simulink model "abslut10_fixpt8_32"  (R2021b)
settings: Solver=VariableStepAuto  StartTime=0.0  StopTime=99  RelTol=1e-3
undefined symbols (not defined in the file or in its folder): figd2104, xcu250
libraries: hdlBasic x2875, vmcUtilities x1
(part 12 of 24)

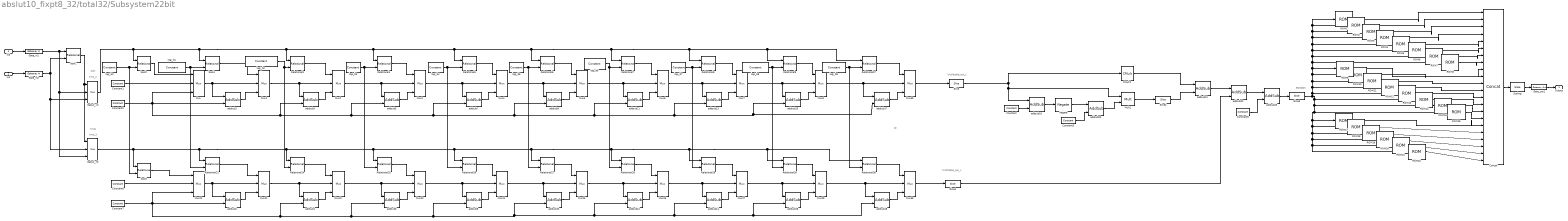
== system abslut10_fixpt8_32/total32/Subsystem22bit ==
  note: 10
  note: tiisai
  note: ooki
  note: 55no6bit
  note: tmp_2
  note: tmp_3
  note: truthtable_out_x
  note: truthtable_out_y
  In3 : Inport
  In4 : Inport  Port=2
  CMult1 : hdlBasic/CMult  const=10  gui_display_data_type=Fixed-point  const_n_bits=4  const_bin_pt=0  float_type=Single  exp_bits=8  fraction_bits=24  en=off  latency=0  precision=Full  arith_type="Signed  (2's comp)"  n_bits=16  bin_pt=14  quantization=Truncate  overflow=Wrap  use_behavioral_HDL=off  mem_type=Distributed RAM  pipeline=off  XmcBlockStatus=1  maskContainerNames=tabcontainer1  block_type=cmult  block_config=sysgen:CMult_config
      settings: infoedit=[]
  Concat : hdlBasic/Concat  num_inputs=22  XmcBlockStatus=1  maskContainerNames=group1  block_type=concat  block_config=sysgen:Concat_config
  Constant : hdlBasic/Constant  const=1.0  gui_display_data_type=Fixed-point  arith_type=Unsigned  n_bits=1  bin_pt=0  preci_type=Single  exp_width=8  frac_width=24  explicit_period=on  period=1  XmcBlockStatus=1  maskContainerNames=tabcontainer1  block_type=constant  block_config=sysgen:Constant_config
  Constant1 : hdlBasic/Constant  const=0  gui_display_data_type=Fixed-point  arith_type=Unsigned  n_bits=4  bin_pt=0  preci_type=Single  exp_width=8  frac_width=24  explicit_period=on  period=1  XmcBlockStatus=1  maskContainerNames=tabcontainer1  block_type=constant  block_config=sysgen:Constant_config
  Constant2 : hdlBasic/Constant  const=1  gui_display_data_type=Fixed-point  arith_type=Unsigned  n_bits=4  bin_pt=0  preci_type=Single  exp_width=8  frac_width=24  explicit_period=on  period=1  XmcBlockStatus=1  maskContainerNames=tabcontainer1  block_type=constant  block_config=sysgen:Constant_config
  Constant3 : hdlBasic/Constant  const=18  gui_display_data_type=Fixed-point  arith_type=Unsigned  n_bits=6  bin_pt=0  preci_type=Single  exp_width=8  frac_width=24  explicit_period=on  period=1  XmcBlockStatus=1  maskContainerNames=tabcontainer1  block_type=constant  block_config=sysgen:Constant_config
  Constant5 : hdlBasic/Constant  const=1.0  gui_display_data_type=Fixed-point  arith_type=Unsigned  n_bits=10  bin_pt=0  preci_type=Single  exp_width=8  frac_width=24  explicit_period=on  period=1  XmcBlockStatus=1  maskContainerNames=tabcontainer1  block_type=constant  block_config=sysgen:Constant_config
  Constant6 : hdlBasic/Constant  const=0  gui_display_data_type=Fixed-point  arith_type=Unsigned  n_bits=4  bin_pt=0  preci_type=Single  exp_width=8  frac_width=24  explicit_period=on  period=1  XmcBlockStatus=1  maskContainerNames=tabcontainer1  block_type=constant  block_config=sysgen:Constant_config
  Constant7 : hdlBasic/Constant  const=1  gui_display_data_type=Fixed-point  arith_type=Unsigned  n_bits=4  bin_pt=0  preci_type=Single  exp_width=8  frac_width=24  explicit_period=on  period=1  XmcBlockStatus=1  maskContainerNames=tabcontainer1  block_type=constant  block_config=sysgen:Constant_config
  Gate_In1 : hdlBasic/Gateway In  gui_display_data_type=Fixed-point  arith_type=Signed (2's comp)  n_bits=22  bin_pt=20  preci_type=Double  exp_width=8  frac_width=24  rows=1  columns=1  quantization="Round  (unbiased: +/- Inf)"  overflow=Saturate  period=1  UseAsADC=off  ADCChannel='1'  interface=None  automatic_assignment=on  address_offset=hex2dec('00')  intf_name=''  intf_description=''  default_value=0  timing_constraint=None  locs_specified=off  LOCs={}  io_standard={}  inherit_from_input=off  hdl_port=on  XmcBlockStatus=1  maskContainerNames=group4  block_type=gatewayin  block_config=sysgen:gateway_in_config  block_width_w=590  block_height_w=620  block_width=640  block_height=850
  Gate_In2 : hdlBasic/Gateway In  gui_display_data_type=Fixed-point  arith_type=Signed (2's comp)  n_bits=22  bin_pt=20  preci_type=Double  exp_width=8  frac_width=24  rows=1  columns=1  quantization="Round  (unbiased: +/- Inf)"  overflow=Saturate  period=1  UseAsADC=off  ADCChannel='1'  interface=None  automatic_assignment=on  address_offset=hex2dec('00')  intf_name=''  intf_description=''  default_value=0  timing_constraint=None  locs_specified=off  LOCs={}  io_standard={}  inherit_from_input=off  hdl_port=on  XmcBlockStatus=1  maskContainerNames=group4  block_type=gatewayin  block_config=sysgen:gateway_in_config  block_width_w=590  block_height_w=620  block_width=640  block_height=850
  Gate_out1 : hdlBasic/Gateway Out  inherit_from_input=off  hdl_port=on  rows=1  columns=1  UseAsDAC=off  DACChannel='1'  interface=None  automatic_assignment=on  address_offset=hex2dec('00')  intf_name=''  intf_description=''  timing_constraint=None  locs_specified=off  LOCs={}  io_standard={}  XmcBlockStatus=1  maskContainerNames=group4  block_type=gatewayout  block_config=sysgen:gateway_out_config  block_width_w=590  block_height_w=620  block_width=620  block_height=750
  Mult1 : hdlBasic/Mult  precision=Full  arith_type="Signed  (2's comp)"  n_bits=30  bin_pt=16  quantization="Round  (unbiased: +/- Inf)"  overflow=Saturate  en=off  latency=0  use_behavioral_HDL=off  opt=Area  use_embedded=off  optimum_pipeline=off  pipeline=on  use_rpm=on  placement_style=Triangular  XmcBlockStatus=1  maskContainerNames=group1  block_type=mult  block_config=sysgen:Mult_config
  Mux{,1..8,20..28,38..39} (20 alike) : hdlBasic/Mux  inputs=2  en=off  latency=0  precision=Full  arith_type=Unsigned  n_bits=16  bin_pt=14  quantization=Truncate  overflow=Wrap  XmcBlockStatus=1  maskContainerNames=tabcontainer1  block_type=mux  block_config=sysgen:Mux_config
  Negate : hdlBasic/Negate  precision=Full  arith_type=Unsigned  n_bits=16  bin_pt=14  quantization=Truncate  overflow=Wrap  en=off  latency=0  XmcBlockStatus=1  maskContainerNames=tabcontainer1  block_type=negate  block_config=sysgen:Negate_config
  ROM1 : hdlBasic/ROM  depth=55  initVector=[1,1,1,1,0,0,1,0,0,0,1,0,0,0,0,1,0,0,0,0,0,1,0,0,0,0,0,0,1,0,0,0,0,0,0,0,1,1,0,0,0,0,0,0,1,1,1,1,1,1,1,1,1,1,1]  distributed_mem=Distributed memory  rst=off  init_reg=0  en=off  latency=0  gui_display_data_type=Boolean  arith_type=Boolean  n_bits=2  bin_pt=0  preci_type=Double  exp_width=8  frac_width=24  optimize=Speed  use_rpm=on  simulation_type=fast_sim  XmcBlockStatus=1  maskContainerNames=tabcontainer1  block_type=sprom  block_config=sysgen:SPROM_config
  ROM10 : hdlBasic/ROM  depth=55  initVector=[0,0,1,1,1,0,1,1,1,1,1,0,0,1,0,1,0,0,1,0,0,1,1,1,1,1,1,1,1,1,0,1,0,0,1,0,0,1,1,1,0,0,1,1,1,0,0,1,1,1,1,1,1,0,0]  distributed_mem=Distributed memory  rst=off  init_reg=0  en=off  latency=0  gui_display_data_type=Boolean  arith_type=Boolean  n_bits=2  bin_pt=0  preci_type=Double  exp_width=8  frac_width=24  optimize=Speed  use_rpm=on  simulation_type=fast_sim  XmcBlockStatus=1  maskContainerNames=tabcontainer1  block_type=sprom  block_config=sysgen:SPROM_config
  ROM11 : hdlBasic/ROM  depth=55  initVector=[0,1,0,1,0,0,1,0,1,0,0,0,0,1,0,0,0,0,1,0,0,1,0,1,0,1,1,0,1,0,0,1,0,0,1,0,1,0,0,0,0,0,0,0,0,0,1,1,1,0,0,1,1,1,0]  distributed_mem=Distributed memory  rst=off  init_reg=0  en=off  latency=0  gui_display_data_type=Boolean  arith_type=Boolean  n_bits=2  bin_pt=0  preci_type=Double  exp_width=8  frac_width=24  optimize=Speed  use_rpm=on  simulation_type=fast_sim  XmcBlockStatus=1  maskContainerNames=tabcontainer1  block_type=sprom  block_config=sysgen:SPROM_config
  ROM12 : hdlBasic/ROM  depth=55  initVector=[0,0,0,0,1,1,0,1,0,1,0,1,0,1,1,0,1,0,1,1,1,0,1,0,1,1,1,1,0,1,1,0,0,0,0,1,0,0,1,1,1,1,1,1,0,0,0,0,0,0,0,0,0,0,0]  distributed_mem=Distributed memory  rst=off  init_reg=0  en=off  latency=0  gui_display_data_type=Boolean  arith_type=Boolean  n_bits=2  bin_pt=0  preci_type=Double  exp_width=8  frac_width=24  optimize=Speed  use_rpm=on  simulation_type=fast_sim  XmcBlockStatus=1  maskContainerNames=tabcontainer1  block_type=sprom  block_config=sysgen:SPROM_config
  ROM13 : hdlBasic/ROM  depth=55  initVector=[0,1,1,1,1,0,1,0,1,0,1,0,0,1,1,1,0,0,1,1,1,1,0,1,0,1,1,0,1,1,0,1,0,0,1,0,1,1,1,0,0,0,0,1,1,0,1,1,1,1,1,1,1,1,0]  distributed_mem=Distributed memory  rst=off  init_reg=0  en=off  latency=0  gui_display_data_type=Boolean  arith_type=Boolean  n_bits=2  bin_pt=0  preci_type=Double  exp_width=8  frac_width=24  optimize=Speed  use_rpm=on  simulation_type=fast_sim  XmcBlockStatus=1  maskContainerNames=tabcontainer1  block_type=sprom  block_config=sysgen:SPROM_config
  ROM14 : hdlBasic/ROM  depth=55  initVector=[1,0,0,1,0,0,1,0,1,1,0,0,1,0,1,0,0,1,0,1,1,1,0,1,1,0,0,1,1,0,0,1,1,1,1,0,0,0,0,0,0,0,0,0,0,1,0,1,1,0,0,1,1,0,1]  distributed_mem=Distributed memory  rst=off  init_reg=0  en=off  latency=0  gui_display_data_type=Boolean  arith_type=Boolean  n_bits=2  bin_pt=0  preci_type=Double  exp_width=8  frac_width=24  optimize=Speed  use_rpm=on  simulation_type=fast_sim  XmcBlockStatus=1  maskContainerNames=tabcontainer1  block_type=sprom  block_config=sysgen:SPROM_config
  ROM15 : hdlBasic/ROM  depth=55  initVector=[0,0,1,0,0,0,0,0,0,1,0,0,0,0,0,0,0,0,0,0,0,0,0,0,1,0,0,1,0,0,0,0,0,0,0,0,0,1,0,0,0,0,0,0,1,0,0,0,0,0,0,0,0,0,0]  distributed_mem=Distributed memory  rst=off  init_reg=0  en=off  latency=0  gui_display_data_type=Boolean  arith_type=Boolean  n_bits=2  bin_pt=0  preci_type=Double  exp_width=8  frac_width=24  optimize=Speed  use_rpm=on  simulation_type=fast_sim  XmcBlockStatus=1  maskContainerNames=tabcontainer1  block_type=sprom  block_config=sysgen:SPROM_config
  ROM16 : hdlBasic/ROM  depth=55  initVector=[0,0,0,1,0,0,0,0,1,0,1,0,0,1,0,1,0,0,1,0,0,0,0,1,0,1,1,0,1,0,0,1,0,0,1,0,0,0,0,0,0,0,0,0,0,0,0,1,0,1,1,0,1,0,0]  distributed_mem=Distributed memory  rst=off  init_reg=0  en=off  latency=0  gui_display_data_type=Boolean  arith_type=Boolean  n_bits=2  bin_pt=0  preci_type=Double  exp_width=8  frac_width=24  optimize=Speed  use_rpm=on  simulation_type=fast_sim  XmcBlockStatus=1  maskContainerNames=tabcontainer1  block_type=sprom  block_config=sysgen:SPROM_config
  ROM17 : hdlBasic/ROM  depth=55  initVector=[1,1,1,0,0,1,1,0,1,1,1,1,1,1,1,1,1,1,1,1,1,1,0,1,1,1,1,1,0,0,1,1,1,1,1,1,1,1,0,0,1,1,0,0,1,1,1,0,1,1,1,1,0,1,1]  distributed_mem=Distributed memory  rst=off  init_reg=0  en=off  latency=0  gui_display_data_type=Boolean  arith_type=Boolean  n_bits=2  bin_pt=0  preci_type=Double  exp_width=8  frac_width=24  optimize=Speed  use_rpm=on  simulation_type=fast_sim  XmcBlockStatus=1  maskContainerNames=tabcontainer1  block_type=sprom  block_config=sysgen:SPROM_config
  ROM18 : hdlBasic/ROM  depth=55  initVector=[1,0,1,0,0,1,0,0,1,1,0,1,1,0,1,0,1,1,0,1,1,0,0,1,1,0,0,1,0,0,1,1,1,1,1,1,0,1,0,0,1,1,0,0,1,1,0,0,0,0,0,0,0,0,1]  distributed_mem=Distributed memory  rst=off  init_reg=0  en=off  latency=0  gui_display_data_type=Boolean  arith_type=Boolean  n_bits=2  bin_pt=0  preci_type=Double  exp_width=8  frac_width=24  optimize=Speed  use_rpm=on  simulation_type=fast_sim  XmcBlockStatus=1  maskContainerNames=tabcontainer1  block_type=sprom  block_config=sysgen:SPROM_config
  ROM19 : hdlBasic/ROM  depth=55  initVector=[1,0,1,1,0,1,0,1,0,1,1,1,1,0,1,1,1,1,0,1,1,0,1,0,1,0,0,1,1,0,1,0,1,1,0,1,0,1,0,1,1,1,1,0,1,1,0,1,0,1,1,0,1,0,1]  distributed_mem=Distributed memory  rst=off  init_reg=0  en=off  latency=0  gui_display_data_type=Boolean  arith_type=Boolean  n_bits=2  bin_pt=0  preci_type=Double  exp_width=8  frac_width=24  optimize=Speed  use_rpm=on  simulation_type=fast_sim  XmcBlockStatus=1  maskContainerNames=tabcontainer1  block_type=sprom  block_config=sysgen:SPROM_config
  ROM2 : hdlBasic/ROM  depth=55  initVector=[0,0,0,0,1,1,0,1,1,0,0,1,1,0,0,0,1,1,0,0,0,0,1,1,0,0,0,0,0,1,1,1,1,1,1,1,0,0,1,1,1,1,1,1,0,0,0,0,0,0,0,0,0,0,0]  distributed_mem=Distributed memory  rst=off  init_reg=0  en=off  latency=0  gui_display_data_type=Boolean  arith_type=Boolean  n_bits=2  bin_pt=0  preci_type=Double  exp_width=8  frac_width=24  optimize=Speed  use_rpm=on  simulation_type=fast_sim  XmcBlockStatus=1  maskContainerNames=tabcontainer1  block_type=sprom  block_config=sysgen:SPROM_config
  ROM20 : hdlBasic/ROM  depth=55  initVector=[1,0,1,1,1,1,0,0,1,1,0,1,1,0,1,0,1,1,0,1,1,0,0,1,1,0,0,1,1,1,1,1,1,1,1,1,0,1,1,0,1,1,0,1,1,1,0,1,0,0,0,0,1,0,1]  distributed_mem=Distributed memory  rst=off  init_reg=0  en=off  latency=0  gui_display_data_type=Boolean  arith_type=Boolean  n_bits=2  bin_pt=0  preci_type=Double  exp_width=8  frac_width=24  optimize=Speed  use_rpm=on  simulation_type=fast_sim  XmcBlockStatus=1  maskContainerNames=tabcontainer1  block_type=sprom  block_config=sysgen:SPROM_config
  ROM21 : hdlBasic/ROM  depth=55  initVector=[0,0,0,1,1,1,0,1,1,1,0,1,0,0,1,0,1,0,0,1,1,0,1,1,1,0,0,1,1,1,1,1,0,0,1,1,0,0,1,1,1,1,1,1,0,0,0,1,0,0,0,0,1,0,0]  distributed_mem=Distributed memory  rst=off  init_reg=0  en=off  latency=0  gui_display_data_type=Boolean  arith_type=Boolean  n_bits=2  bin_pt=0  preci_type=Double  exp_width=8  frac_width=24  optimize=Speed  use_rpm=on  simulation_type=fast_sim  XmcBlockStatus=1  maskContainerNames=tabcontainer1  block_type=sprom  block_config=sysgen:SPROM_config
  ROM22 : hdlBasic/ROM  depth=55  initVector=[0,1,1,1,1,0,0,1,0,0,1,0,1,0,1,1,0,1,0,1,1,0,1,0,0,0,0,0,1,1,0,0,1,1,0,0,1,1,1,1,0,0,1,1,1,0,1,1,0,1,1,0,1,1,0]  distributed_mem=Distributed memory  rst=off  init_reg=0  en=off  latency=0  gui_display_data_type=Boolean  arith_type=Boolean  n_bits=2  bin_pt=0  preci_type=Double  exp_width=8  frac_width=24  optimize=Speed  use_rpm=on  simulation_type=fast_sim  XmcBlockStatus=1  maskContainerNames=tabcontainer1  block_type=sprom  block_config=sysgen:SPROM_config
  ROM3 : hdlBasic/ROM  depth=55  initVector=[1,1,0,0,1,1,0,1,0,1,0,1,0,1,0,0,1,0,1,0,0,0,1,0,1,1,1,1,0,1,1,0,0,0,0,1,1,0,1,1,1,1,1,1,0,1,1,0,0,0,0,0,0,1,1]  distributed_mem=Distributed memory  rst=off  init_reg=0  en=off  latency=0  gui_display_data_type=Boolean  arith_type=Boolean  n_bits=2  bin_pt=0  preci_type=Double  exp_width=8  frac_width=24  optimize=Speed  use_rpm=on  simulation_type=fast_sim  XmcBlockStatus=1  maskContainerNames=tabcontainer1  block_type=sprom  block_config=sysgen:SPROM_config
  ROM4 : hdlBasic/ROM  depth=55  initVector=[1,0,0,1,1,0,0,0,1,1,0,0,0,0,1,0,0,0,0,1,1,0,0,1,1,0,0,1,1,1,0,1,0,0,1,0,0,0,1,0,0,0,0,1,0,1,0,1,0,0,0,0,1,0,1]  distributed_mem=Distributed memory  rst=off  init_reg=0  en=off  latency=0  gui_display_data_type=Boolean  arith_type=Boolean  n_bits=2  bin_pt=0  preci_type=Double  exp_width=8  frac_width=24  optimize=Speed  use_rpm=on  simulation_type=fast_sim  XmcBlockStatus=1  maskContainerNames=tabcontainer1  block_type=sprom  block_config=sysgen:SPROM_config
  ROM5 : hdlBasic/ROM  depth=55  initVector=[0,0,1,0,1,0,0,1,0,1,0,0,1,1,0,0,0,1,1,0,0,0,1,0,1,1,1,1,0,1,0,0,1,1,0,0,0,1,1,1,0,0,1,1,1,0,0,0,0,0,0,0,0,0,0]  distributed_mem=Distributed memory  rst=off  init_reg=0  en=off  latency=0  gui_display_data_type=Boolean  arith_type=Boolean  n_bits=2  bin_pt=0  preci_type=Double  exp_width=8  frac_width=24  optimize=Speed  use_rpm=on  simulation_type=fast_sim  XmcBlockStatus=1  maskContainerNames=tabcontainer1  block_type=sprom  block_config=sysgen:SPROM_config
  ROM6 : hdlBasic/ROM  depth=55  initVector=[1,0,1,0,0,1,1,1,0,1,0,1,0,1,1,0,1,0,1,1,1,1,1,0,1,1,1,1,0,0,1,0,0,0,0,1,0,1,0,1,1,1,1,0,1,1,0,0,1,0,0,1,0,0,1]  distributed_mem=Distributed memory  rst=off  init_reg=0  en=off  latency=0  gui_display_data_type=Boolean  arith_type=Boolean  n_bits=2  bin_pt=0  preci_type=Double  exp_width=8  frac_width=24  optimize=Speed  use_rpm=on  simulation_type=fast_sim  XmcBlockStatus=1  maskContainerNames=tabcontainer1  block_type=sprom  block_config=sysgen:SPROM_config
  ROM7 : hdlBasic/ROM  depth=55  initVector=[0,1,0,1,1,0,1,0,1,0,0,0,0,0,0,0,0,0,0,0,0,1,0,1,0,0,0,0,1,1,0,1,0,0,1,0,1,0,1,0,0,0,0,1,0,0,1,1,1,0,0,1,1,1,0]  distributed_mem=Distributed memory  rst=off  init_reg=0  en=off  latency=0  gui_display_data_type=Boolean  arith_type=Boolean  n_bits=2  bin_pt=0  preci_type=Double  exp_width=8  frac_width=24  optimize=Speed  use_rpm=on  simulation_type=fast_sim  XmcBlockStatus=1  maskContainerNames=tabcontainer1  block_type=sprom  block_config=sysgen:SPROM_config
  ROM8 : hdlBasic/ROM  depth=55  initVector=[1,0,0,0,0,0,0,0,0,0,0,0,0,0,0,0,0,0,0,0,0,0,0,0,0,0,0,0,0,0,0,0,0,0,0,0,0,0,0,0,0,0,0,0,0,1,0,0,0,0,0,0,0,0,1]  distributed_mem=Distributed memory  rst=off  init_reg=0  en=off  latency=0  gui_display_data_type=Boolean  arith_type=Boolean  n_bits=2  bin_pt=0  preci_type=Double  exp_width=8  frac_width=24  optimize=Speed  use_rpm=on  simulation_type=fast_sim  XmcBlockStatus=1  maskContainerNames=tabcontainer1  block_type=sprom  block_config=sysgen:SPROM_config
  ROM9 : hdlBasic/ROM  depth=55  initVector=[0,0,1,0,0,1,1,0,1,0,1,1,1,1,0,1,1,1,1,0,0,1,0,1,0,1,1,0,0,0,1,1,1,1,1,1,0,1,0,0,1,1,0,0,1,0,0,0,1,1,1,1,0,0,0]  distributed_mem=Distributed memory  rst=off  init_reg=0  en=off  latency=0  gui_display_data_type=Boolean  arith_type=Boolean  n_bits=2  bin_pt=0  preci_type=Double  exp_width=8  frac_width=24  optimize=Speed  use_rpm=on  simulation_type=fast_sim  XmcBlockStatus=1  maskContainerNames=tabcontainer1  block_type=sprom  block_config=sysgen:SPROM_config
  Relational{3..9,21,24..30,37..38} (17 alike) : hdlBasic/Relational  mode=a>=b  op_type=Bool  en=off  latency=0  XmcBlockStatus=1  maskContainerNames=tabcontainer1  block_type=relational  block_config=sysgen:Relational_config
  Scaling : hdlBasic/Scale  scale_factor=-21  XmcBlockStatus=1  maskContainerNames=group1  block_type=scale  block_config=sysgen:Scale_config
  Slice : hdlBasic/Slice  nbits=4  boolean_output=off  mode=Lower Bit Location + Width  bit1=-1  base1=MSB of Input  bit0=0  base0=LSB of Input  XmcBlockStatus=1  maskContainerNames=group1  block_type=slice  block_config=sysgen:Slice_config
  Slice1 : hdlBasic/Slice  nbits=4  boolean_output=off  mode=Lower Bit Location + Width  bit1=-1  base1=MSB of Input  bit0=0  base0=LSB of Input  XmcBlockStatus=1  maskContainerNames=group1  block_type=slice  block_config=sysgen:Slice_config
  Slice2 : hdlBasic/Slice  nbits=21  boolean_output=off  mode=Two Bit Locations  bit1=-1  base1=MSB of Input  bit0=1  base0=LSB of Input  XmcBlockStatus=1  maskContainerNames=group1  block_type=slice  block_config=sysgen:Slice_config
  Slice3 : hdlBasic/Slice  nbits=21  boolean_output=off  mode=Two Bit Locations  bit1=-5  base1=MSB of Input  bit0=0  base0=LSB of Input  XmcBlockStatus=1  maskContainerNames=group1  block_type=slice  block_config=sysgen:Slice_config
  addsub{1..18} (18 alike) : hdlBasic/AddSub  mode=Addition  use_carryin=off  use_carryout=off  en=off  latency=0  precision=User Defined  arith_type=Unsigned  n_bits=4  bin_pt=0  quantization="Round  (unbiased: +/- Inf)"  overflow=Saturate  use_behavioral_HDL=off  hw_selection=Fabric  pipelined=on  XmcBlockStatus=1  maskContainerNames=tabcontainer1  block_type=addsub  block_config=sysgen:Addsub_config
  addsub19 : hdlBasic/AddSub  mode=Subtraction  use_carryin=off  use_carryout=off  en=off  latency=0  precision=Full  arith_type=Unsigned  n_bits=5  bin_pt=0  quantization=Truncate  overflow=Wrap  use_behavioral_HDL=off  hw_selection=Fabric  pipelined=on  XmcBlockStatus=1  maskContainerNames=tabcontainer1  block_type=addsub  block_config=sysgen:Addsub_config
  addsub20 : hdlBasic/AddSub  mode=Addition  use_carryin=off  use_carryout=off  en=off  latency=0  precision=Full  arith_type=Unsigned  n_bits=16  bin_pt=14  quantization=Truncate  overflow=Wrap  use_behavioral_HDL=off  hw_selection=Fabric  pipelined=on  XmcBlockStatus=1  maskContainerNames=tabcontainer1  block_type=addsub  block_config=sysgen:Addsub_config
  addsub21 : hdlBasic/AddSub  mode=Subtraction  use_carryin=off  use_carryout=off  en=off  latency=0  precision=User Defined  arith_type=Unsigned  n_bits=6  bin_pt=0  quantization="Round  (unbiased: +/- Inf)"  overflow=Saturate  use_behavioral_HDL=off  hw_selection=Fabric  pipelined=on  XmcBlockStatus=1  maskContainerNames=tabcontainer1  block_type=addsub  block_config=sysgen:Addsub_config
  addsub22 : hdlBasic/AddSub  mode=Addition  use_carryin=off  use_carryout=off  en=off  latency=0  precision=Full  arith_type=Unsigned  n_bits=16  bin_pt=14  quantization=Truncate  overflow=Wrap  use_behavioral_HDL=off  hw_selection=Fabric  pipelined=on  XmcBlockStatus=1  maskContainerNames=tabcontainer1  block_type=addsub  block_config=sysgen:Addsub_config
  addsub23 : hdlBasic/AddSub  mode=Subtraction  use_carryin=off  use_carryout=off  en=off  latency=0  precision=Full  arith_type=Unsigned  n_bits=6  bin_pt=0  quantization=Truncate  overflow=Wrap  use_behavioral_HDL=off  hw_selection=Fabric  pipelined=on  XmcBlockStatus=1  maskContainerNames=tabcontainer1  block_type=addsub  block_config=sysgen:Addsub_config
  bool1 : hdlBasic/Relational  mode=a<b  op_type=Bool  en=off  latency=0  XmcBlockStatus=1  maskContainerNames=tabcontainer1  block_type=relational  block_config=sysgen:Relational_config
  bool2 : hdlBasic/Relational  mode=a>=b  op_type=Bool  en=off  latency=0  XmcBlockStatus=1  maskContainerNames=tabcontainer1  block_type=relational  block_config=sysgen:Relational_config
  bool3 : hdlBasic/Relational  mode=a>=b  op_type=Bool  en=off  latency=0  XmcBlockStatus=1  maskContainerNames=tabcontainer1  block_type=relational  block_config=sysgen:Relational_config
  bool4 : hdlBasic/Relational  mode=a>=b  op_type=Bool  en=off  latency=0  XmcBlockStatus=1  maskContainerNames=tabcontainer1  block_type=relational  block_config=sysgen:Relational_config
  logi_b0 : hdlBasic/Constant  const=-1.0000000000000000000000000000000000000000000000000000000  gui_display_data_type=Fixed-point  arith_type=Signed (2's comp)  n_bits=22  bin_pt=21  preci_type=Double  exp_width=8  frac_width=24  explicit_period=on  period=1  XmcBlockStatus=1  maskContainerNames=tabcontainer1  block_type=constant  block_config=sysgen:Constant_config
  logi_b1 : hdlBasic/Constant  const=-0.7777777777777776790912866999860852956771850585937500000  gui_display_data_type=Fixed-point  arith_type=Signed (2's comp)  n_bits=22  bin_pt=21  preci_type=Double  exp_width=8  frac_width=24  explicit_period=on  period=1  XmcBlockStatus=1  maskContainerNames=tabcontainer1  block_type=constant  block_config=sysgen:Constant_config
  logi_b2 : hdlBasic/Constant  const=-0.5555555555555555802271783250034786760807037353515625000  gui_display_data_type=Fixed-point  arith_type=Signed (2's comp)  n_bits=22  bin_pt=21  preci_type=Double  exp_width=8  frac_width=24  explicit_period=on  period=1  XmcBlockStatus=1  maskContainerNames=tabcontainer1  block_type=constant  block_config=sysgen:Constant_config
  logi_b3 : hdlBasic/Constant  const=-0.3333333333333333148296162562473909929394721984863281250  gui_display_data_type=Fixed-point  arith_type=Signed (2's comp)  n_bits=22  bin_pt=21  preci_type=Double  exp_width=8  frac_width=24  explicit_period=on  period=1  XmcBlockStatus=1  maskContainerNames=tabcontainer1  block_type=constant  block_config=sysgen:Constant_config
  logi_b4 : hdlBasic/Constant  const=-0.1111111111111111049432054187491303309798240661621093750  gui_display_data_type=Fixed-point  arith_type=Signed (2's comp)  n_bits=22  bin_pt=21  preci_type=Double  exp_width=8  frac_width=24  explicit_period=on  period=1  XmcBlockStatus=1  maskContainerNames=tabcontainer1  block_type=constant  block_config=sysgen:Constant_config
  logi_b5 : hdlBasic/Constant  const=0.1111111111111111049432054187491303309798240661621093750  gui_display_data_type=Fixed-point  arith_type=Signed (2's comp)  n_bits=22  bin_pt=21  preci_type=Double  exp_width=8  frac_width=24  explicit_period=on  period=1  XmcBlockStatus=1  maskContainerNames=tabcontainer1  block_type=constant  block_config=sysgen:Constant_config
  logi_b6 : hdlBasic/Constant  const=0.3333333333333333148296162562473909929394721984863281250  gui_display_data_type=Fixed-point  arith_type=Signed (2's comp)  n_bits=22  bin_pt=21  preci_type=Double  exp_width=8  frac_width=24  explicit_period=on  period=1  XmcBlockStatus=1  maskContainerNames=tabcontainer1  block_type=constant  block_config=sysgen:Constant_config
  logi_b7 : hdlBasic/Constant  const=0.5555555555555555802271783250034786760807037353515625000  gui_display_data_type=Fixed-point  arith_type=Signed (2's comp)  n_bits=22  bin_pt=21  preci_type=Double  exp_width=8  frac_width=24  explicit_period=on  period=1  XmcBlockStatus=1  maskContainerNames=tabcontainer1  block_type=constant  block_config=sysgen:Constant_config
  logi_b8 : hdlBasic/Constant  const=0.7777777777777776790912866999860852956771850585937500000  gui_display_data_type=Fixed-point  arith_type=Signed (2's comp)  n_bits=22  bin_pt=21  preci_type=Double  exp_width=8  frac_width=24  explicit_period=on  period=1  XmcBlockStatus=1  maskContainerNames=tabcontainer1  block_type=constant  block_config=sysgen:Constant_config
  logi_b9 : hdlBasic/Constant  const=1.0000000000000000000000000000000000000000000000000000000  gui_display_data_type=Fixed-point  arith_type=Signed (2's comp)  n_bits=22  bin_pt=21  preci_type=Double  exp_width=8  frac_width=24  explicit_period=on  period=1  XmcBlockStatus=1  maskContainerNames=tabcontainer1  block_type=constant  block_config=sysgen:Constant_config
  logical_x0 : hdlBasic/Mux  inputs=2  en=off  latency=0  precision=Full  arith_type=Unsigned  n_bits=16  bin_pt=14  quantization=Truncate  overflow=Wrap  XmcBlockStatus=1  maskContainerNames=tabcontainer1  block_type=mux  block_config=sysgen:Mux_config
  logical_y0 : hdlBasic/Mux  inputs=2  en=off  latency=0  precision=Full  arith_type=Unsigned  n_bits=16  bin_pt=14  quantization=Truncate  overflow=Wrap  XmcBlockStatus=1  maskContainerNames=tabcontainer1  block_type=mux  block_config=sysgen:Mux_config
  Output : Outport
  wires:
  addsub9/1 -> Mux5/3
  In4/1 -> Gate_In2/1
  addsub13/1 -> Mux7/3
  In3/1 -> Gate_In1/1
  addsub1/1 -> Mux1/3
  addsub5/1 -> Mux3/3
  addsub3/1 -> Mux2/3
  bool2/1 -> Mux/1
  addsub7/1 -> Mux4/3
  addsub11/1 -> Mux6/3
  addsub15/1 -> Mux8/3
  bool1/1 -> logical_x0/1, logical_y0/1
  Constant3/1 -> addsub20/2
  Constant/1 -> addsub19/2
  addsub20/1 -> Mult1/2
  addsub19/1 -> Negate/1
  addsub23/1 -> Slice3/1
  addsub22/1 -> addsub23/1
  addsub21/1 -> addsub22/1
  CMult1/1 -> addsub21/1
  Negate/1 -> addsub20/1
  Mult1/1 -> Slice2/1
  Gate_In2/1 -> bool1/2, logical_x0/2, logical_y0/3
  Gate_In1/1 -> bool1/1, logical_x0/3, logical_y0/2
  bool4/1 -> Mux1/1
  Mux/1 -> Mux1/2, addsub1/1
  Relational3/1 -> Mux2/1
  Mux1/1 -> Mux2/2, addsub3/1
  Relational4/1 -> Mux3/1
  Mux2/1 -> Mux3/2, addsub5/1
  Relational5/1 -> Mux4/1
  Mux3/1 -> Mux4/2, addsub7/1
  Relational6/1 -> Mux5/1
  Mux4/1 -> Mux5/2, addsub9/1
  Relational7/1 -> Mux6/1
  Mux5/1 -> Mux6/2, addsub11/1
  Relational8/1 -> Mux7/1
  Mux6/1 -> Mux7/2, addsub13/1
  Relational9/1 -> Mux8/1
  Mux7/1 -> Mux8/2, addsub15/1
  Mux21/1 -> Mux22/2, addsub4/1
  Mux26/1 -> Mux27/2, addsub14/1
  Relational30/1 -> Mux28/1
  Relational26/1 -> Mux24/1
  logi_b3/1 -> Relational25/2, Relational4/2
  addsub4/1 -> Mux22/3
  addsub12/1 -> Mux26/3
  Relational27/1 -> Mux25/1
  logi_b1/1 -> Relational21/2, bool4/2
  bool3/1 -> Mux20/1
  addsub6/1 -> Mux23/3
  Mux22/1 -> Mux23/2, addsub6/1
  Relational28/1 -> Mux26/1
  logi_b4/1 -> Relational26/2, Relational5/2
  Mux23/1 -> Mux24/2, addsub8/1
  logi_b7/1 -> Relational29/2, Relational8/2
  Relational29/1 -> Mux27/1
  logi_b0/1 -> bool3/2, bool2/2
  Mux27/1 -> Mux28/2, addsub16/1
  logi_b5/1 -> Relational27/2, Relational6/2
  Mux20/1 -> Mux21/2, addsub2/1
  Relational25/1 -> Mux23/1
  Mux25/1 -> Mux26/2, addsub12/1
  Relational24/1 -> Mux22/1
  logi_b2/1 -> Relational3/2, Relational24/2
  addsub8/1 -> Mux24/3
  addsub14/1 -> Mux27/3
  Mux24/1 -> Mux25/2, addsub10/1
  logi_b6/1 -> Relational28/2, Relational7/2
  Relational21/1 -> Mux21/1
  addsub10/1 -> Mux25/3
  addsub16/1 -> Mux28/3
  logi_b8/1 -> Relational30/2, Relational9/2
  addsub2/1 -> Mux21/3
  Constant6/1 -> Mux20/2
  Constant1/1 -> Mux/2
  Slice/1 -> CMult1/1, Mult1/1, addsub19/1
  Slice1/1 -> addsub22/2
  Mux8/1 -> Mux39/2, addsub17/1
  logi_b9/1 -> Relational38/2, Relational37/2
  Relational37/1 -> Mux39/1
  addsub18/1 -> Mux38/3
  Relational38/1 -> Mux38/1
  Constant7/1 -> addsub18/2, addsub16/2, addsub14/2, addsub12/2, addsub10/2, addsub8/2, addsub6/2, addsub4/2, addsub2/2, Mux20/3
  Constant2/1 -> addsub17/2, addsub15/2, addsub13/2, addsub11/2, addsub9/2, addsub7/2, addsub5/2, addsub3/2, addsub1/2, Mux/3
  addsub17/1 -> Mux39/3
  Mux28/1 -> Mux38/2, addsub18/1
  Mux39/1 -> Slice/1
  Mux38/1 -> Slice1/1
  Gate_out1/1 -> Output/1
  Slice2/1 -> addsub21/2
  Constant5/1 -> addsub23/2
  logical_y0/1 -> Relational37/1, Relational9/1, Relational8/1, Relational7/1, Relational6/1, Relational5/1, Relational4/1, Relational3/1, bool4/1, bool2/1
  logical_x0/1 -> Relational38/1, Relational30/1, Relational29/1, Relational28/1, Relational27/1, Relational26/1, Relational25/1, Relational24/1, Relational21/1, bool3/1
  Concat/1 -> Scaling/1
  Scaling/1 -> Gate_out1/1
  ROM1/1 -> Concat/1
  ROM14/1 -> Concat/14
  ROM8/1 -> Concat/8
  ROM9/1 -> Concat/9
  ROM21/1 -> Concat/21
  ROM11/1 -> Concat/11
  ROM18/1 -> Concat/18
  ROM22/1 -> Concat/22
  ROM20/1 -> Concat/20
  ROM2/1 -> Concat/2
  ROM13/1 -> Concat/13
  Slice3/1 -> ROM13/1, ROM12/1, ROM11/1, ROM10/1, ROM9/1, ROM4/1, ROM1/1, ROM2/1, ROM3/1, ROM5/1, ROM6/1, ROM7/1, ROM8/1, ROM22/1, ROM21/1, ROM20/1, ROM19/1, ROM18/1, ROM17/1, ROM16/1, ROM15/1, ROM14/1
  ROM19/1 -> Concat/19
  ROM16/1 -> Concat/16
  ROM4/1 -> Concat/4
  ROM5/1 -> Concat/5
  ROM10/1 -> Concat/10
  ROM7/1 -> Concat/7
  ROM6/1 -> Concat/6
  ROM15/1 -> Concat/15
  ROM12/1 -> Concat/12
  ROM3/1 -> Concat/3
  ROM17/1 -> Concat/17
